simulink model "adaptivekoli"  (Simulink 7.1)
settings: Solver=ode45  StartTime=0.0  StopTime=100  RelTol=1e-3
InitFcn:
  | vo=502;
  | za=-1.01887*502;
  | zq=0.0949*502;
  | zd=-0.00215*502;
  | ma=0.82225;
  | mq=-1.07741;
  | md=-0.17555;
settings Model: Creator=zahra yaghoubi  LastModifiedBy=Yaghobi
settings OptimizationCC: InitFltsAndDblsToZero=off
settings DebuggingCC: StrictBusMsg=ErrorLevel1

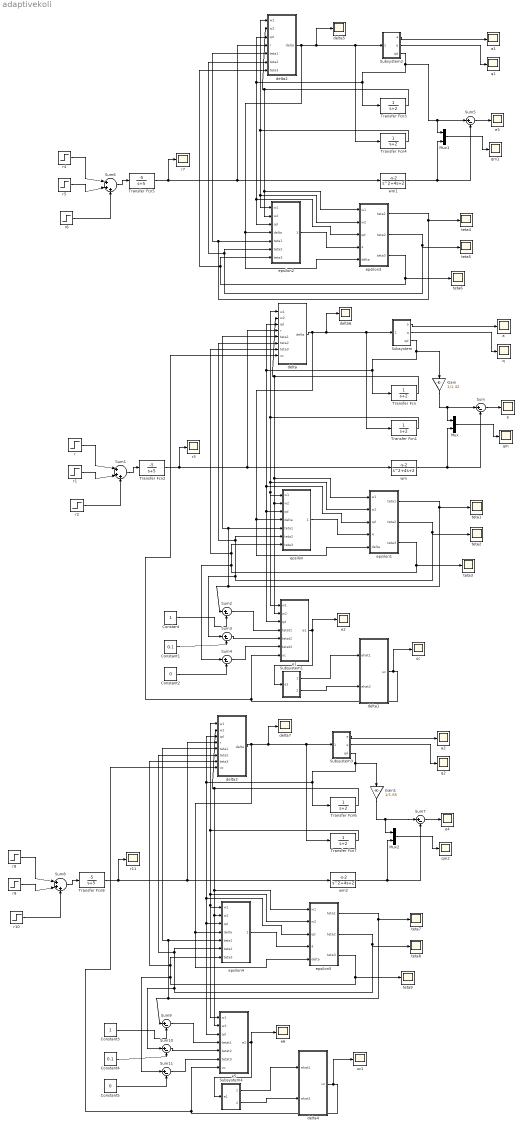
== system adaptivekoli ==
  Constant : Constant  OutDataType=sfix(16)  OutScaling=2^0
  Constant1 : Constant  Value=0.1  OutDataType=sfix(16)  OutScaling=2^0
  Constant2 : Constant  Value=0  OutDataType=sfix(16)  OutScaling=2^0
  Constant3 : Constant  OutDataType=sfix(16)  OutScaling=2^0
  Constant4 : Constant  Value=0.1  OutDataType=sfix(16)  OutScaling=2^0
  Constant5 : Constant  Value=0  OutDataType=sfix(16)  OutScaling=2^0
  Gain : Gain  Orientation=down  Gain=1/1.42  ParameterDataType=sfix(16)  ParameterScaling=2^0  OutDataType=sfix(16)  OutScaling=2^0
  Gain1 : Gain  Orientation=down  Gain=1/1.65  ParameterDataType=sfix(16)  ParameterScaling=2^0  OutDataType=sfix(16)  OutScaling=2^0
  Mux : Mux  Inputs=2
  Mux1 : Mux  Inputs=2
  Mux2 : Mux  Inputs=2
  Subsystem : Subsystem
  Subsystem1 : Subsystem
  Subsystem2 : Subsystem
  Subsystem3 : Subsystem
  Subsystem4 : Subsystem
  Sum{,2..5,7,9..11} (9 alike) : Sum  Inputs=|+-  OutDataType=sfix(16)  OutScaling=2^0
  Sum1 : Sum  Inputs=|+++  OutDataType=sfix(16)  OutScaling=2^0
  Sum6 : Sum  Inputs=|+++  OutDataType=sfix(16)  OutScaling=2^0
  Sum8 : Sum  Inputs=|+++  OutDataType=sfix(16)  OutScaling=2^0
  Transfer Fcn{,1,3..4,6..7} (6 alike) : TransferFcn  Denominator=[1 2]
  Transfer Fcn2 : TransferFcn  Numerator=[-5]  Denominator=[1 5]
  Transfer Fcn5 : TransferFcn  Numerator=[-5]  Denominator=[1 5]
  Transfer Fcn8 : TransferFcn  Numerator=[-5]  Denominator=[1 5]
  a : Scope
      settings: SaveName=a2  DataFormat=Array  MaxDataPoints=50000
  a1 : Scope
      settings: SaveName=a1  DataFormat=Array  MaxDataPoints=50000
  a2 : Scope
      settings: SaveName=a3  DataFormat=Array  MaxDataPoints=50000
  delta : Subsystem
  delta1 : Subsystem
  delta2 : Subsystem
  delta3 : Subsystem
  delta4 : Subsystem
  delta5 : Scope
      settings: SaveName=delta1  DataFormat=Array  MaxDataPoints=50000
  delta6 : Scope
      settings: SaveName=delta2  DataFormat=Array  MaxDataPoints=50000
  delta7 : Scope
      settings: SaveName=delta3  DataFormat=Array  MaxDataPoints=50000
  e{,2..4,6} (5 alike) : Scope
      e settings: SaveName=e2  DataFormat=Array  MaxDataPoints=50000
      e2 settings: MaxDataPoints=50000
      e3 settings: SaveName=e1  DataFormat=Array  MaxDataPoints=50000
      e4 settings: SaveName=e3  DataFormat=Array  MaxDataPoints=50000
      e6 settings: SaveName=ScopeData3  MaxDataPoints=50000
  e1 : Subsystem
  e5 : Subsystem
  epsilon : Subsystem
  epsilon1 : Subsystem
  epsilon2 : Subsystem
  epsilon3 : Subsystem
  epsilon4 : Subsystem
  epsilon5 : Subsystem
  q : Scope
      settings: SaveName=q2  DataFormat=Array  MaxDataPoints=50000
  q1 : Scope
      settings: SaveName=q1  DataFormat=Array  MaxDataPoints=50000
  q2 : Scope
      settings: SaveName=q3  DataFormat=Array  MaxDataPoints=50000
  qm : Scope
      settings: SaveName=qm2  DataFormat=Array  MaxDataPoints=500000
  qm1 : Scope
      settings: SaveName=qm1  DataFormat=Array  MaxDataPoints=500000
  qm2 : Scope
      settings: SaveName=qm3  DataFormat=Array  MaxDataPoints=50000
  r : Step  Time=0  After=-1  SampleTime=0
  r1 : Step  Time=20  After=3  SampleTime=0
  r10 : Step  Time=40  After=-6  SampleTime=0
  r11 : Scope
      settings: SaveName=ScopeData4
  r2 : Step  Time=40  After=-6  SampleTime=0
  r3 : Scope
      settings: SaveName=r  DataFormat=Array  MaxDataPoints=50000
  r4 : Step  Time=0  After=-1  SampleTime=0
  r5 : Step  Time=20  After=3  SampleTime=0
  r6 : Step  Time=40  After=-6  SampleTime=0
  r7 : Scope
      settings: SaveName=ScopeData2
  r8 : Step  Time=0  After=-1  SampleTime=0
  r9 : Step  Time=20  After=3  SampleTime=0
  teta{1..9} (9 alike) : Scope
      teta1 settings: TimeRange=60  YMin=0  YMax=2  SaveName=teta12  DataFormat=Array  MaxDataPoints=50000
      teta2 settings: SaveName=teta22  DataFormat=Array  MaxDataPoints=50000
      teta3 settings: SaveName=teta32  DataFormat=Array  MaxDataPoints=50000
      teta4 settings: SaveName=teta11  DataFormat=Array  MaxDataPoints=50000
      teta5 settings: SaveName=teta21  DataFormat=Array  MaxDataPoints=50000
      teta6 settings: SaveName=teta31  DataFormat=Array  MaxDataPoints=50000
      teta7 settings: TimeRange=60  YMin=0  YMax=2  SaveName=teta13  DataFormat=Array  MaxDataPoints=50000
      teta8 settings: SaveName=teta23  DataFormat=Array  MaxDataPoints=50000
      teta9 settings: SaveName=teta33  DataFormat=Array  MaxDataPoints=50000
  uc : Scope
      settings: SaveName=uc1  DataFormat=Array  MaxDataPoints=50000
  uc1 : Scope
      settings: SaveName=uc2  DataFormat=Array  MaxDataPoints=50000
  wm : TransferFcn  Numerator=[-1 -2]  Denominator="[1 4  2]"
  wm1 : TransferFcn  Numerator=[-1 -2]  Denominator="[1 4  2]"
  wm2 : TransferFcn  Numerator=[-1 -2]  Denominator="[1 4  2]"
  wires:
  Subsystem/1(a) -> a/1
  Subsystem/2(q) -> q/1
  Subsystem/3(qd) -> Transfer Fcn/1, delta/3(qd), epsilon1/3(qd), epsilon/3(qd), e1/3(qd), Gain/1
  delta/1(delta) -> epsilon/4(delta), epsilon1/5(delta), Subsystem/1(delta), Transfer Fcn1/1, delta6/1
  wm/1 -> Sum/2, Mux/2
  Transfer Fcn/1 -> delta/2(w2), epsilon1/1(w1), epsilon/2(w2), e1/2(w2)
  Transfer Fcn1/1 -> delta/1(w1), epsilon1/2(w2), epsilon/1(w1), e1/1(w1)
  epsilon/1(epsilon) -> epsilon1/4(epsilon)
  epsilon1/1(teta1) -> teta1/1, epsilon/5(teta1), delta/5(teta1), Sum2/1
  epsilon1/2(teta2) -> teta2/1, epsilon/6(teta2), delta/6(teta2), Sum3/1
  epsilon1/3(teta3) -> teta3/1, epsilon/7(teta3), delta/7(teta3), Sum4/1
  Sum/1 -> e/1
  r/1 -> Sum1/1
  r1/1 -> Sum1/2
  r2/1 -> Sum1/3
  Sum1/1 -> Transfer Fcn2/1
  Mux/1 -> qm/1
  e1/1(e1) -> Subsystem1/1(e1), e2/1
  Subsystem1/1(ehat1) -> delta1/1(ehat1)
  delta1/1(uc) -> e1/7(uc), delta/8(uc), uc/1
  Sum4/1 -> e1/6(tetat3)
  Sum3/1 -> e1/5(tetat2)
  Sum2/1 -> e1/4(tetat1)
  Constant/1 -> Sum2/2
  Constant1/1 -> Sum3/2
  Constant2/1 -> Sum4/2
  Subsystem1/2(ehat2) -> delta1/2(ehat2)
  Transfer Fcn2/1 -> wm/1, delta/4(r), r3/1
  Gain/1 -> Sum/1, Mux/1
  Subsystem2/1(a) -> a1/1
  Subsystem2/2(q) -> q1/1
  Subsystem2/3(qd) -> Transfer Fcn3/1, delta2/3(qd), epsilon2/3(qd), epsilon3/3(qd), Sum5/1, Mux1/1
  delta2/1(delta) -> epsilon2/4(delta), epsilon3/5(delta), Subsystem2/1(delta), Transfer Fcn4/1, delta5/1
  wm1/1 -> Sum5/2, Mux1/2
  Transfer Fcn3/1 -> delta2/2(w2), epsilon2/2(w2), epsilon3/1(w1)
  Transfer Fcn4/1 -> delta2/1(w1), epsilon2/1(w1), epsilon3/2(w2)
  epsilon2/1(epsilon) -> epsilon3/4(epsilon)
  epsilon3/1(teta1) -> epsilon2/5(teta1), delta2/5(teta1), teta4/1
  epsilon3/2(teta2) -> epsilon2/6(teta2), delta2/6(teta2), teta5/1
  epsilon3/3(teta3) -> epsilon2/7(teta3), delta2/7(teta3), teta6/1
  Sum5/1 -> e3/1
  r4/1 -> Sum6/1
  r5/1 -> Sum6/2
  r6/1 -> Sum6/3
  Sum6/1 -> Transfer Fcn5/1
  Transfer Fcn5/1 -> wm1/1, delta2/4(r), r7/1
  Mux1/1 -> qm1/1
  Subsystem3/1(a) -> a2/1
  Subsystem3/2(q) -> q2/1
  Subsystem3/3(qd) -> Transfer Fcn6/1, delta3/3(qd), epsilon5/3(qd), epsilon4/3(qd), e5/3(qd), Gain1/1
  delta3/1(delta) -> epsilon4/4(delta), epsilon5/5(delta), Subsystem3/1(delta), Transfer Fcn7/1, delta7/1
  wm2/1 -> Sum7/2, Mux2/2
  Transfer Fcn6/1 -> delta3/2(w2), epsilon5/1(w1), epsilon4/2(w2), e5/2(w2)
  Transfer Fcn7/1 -> delta3/1(w1), epsilon5/2(w2), epsilon4/1(w1), e5/1(w1)
  epsilon4/1(epsilon) -> epsilon5/4(epsilon)
  epsilon5/1(teta1) -> teta7/1, epsilon4/5(teta1), delta3/5(teta1), Sum9/1
  epsilon5/2(teta2) -> teta8/1, epsilon4/6(teta2), delta3/6(teta2), Sum10/1
  epsilon5/3(teta3) -> teta9/1, epsilon4/7(teta3), delta3/7(teta3), Sum11/1
  Sum7/1 -> e4/1
  r8/1 -> Sum8/1
  r9/1 -> Sum8/2
  r10/1 -> Sum8/3
  Sum8/1 -> Transfer Fcn8/1
  Mux2/1 -> qm2/1
  e5/1(e1) -> Subsystem4/1(e1), e6/1
  Subsystem4/1(ehat1) -> delta4/1(ehat1)
  delta4/1(uc) -> e5/7(uc), delta3/8(uc), uc1/1
  Sum11/1 -> e5/6(tetat3)
  Sum10/1 -> e5/5(tetat2)
  Sum9/1 -> e5/4(tetat1)
  Constant3/1 -> Sum9/2
  Constant4/1 -> Sum10/2
  Constant5/1 -> Sum11/2
  Subsystem4/2(ehat2) -> delta4/2(ehat2)
  Transfer Fcn8/1 -> wm2/1, delta3/4(r), r11/1
  Gain1/1 -> Sum7/1, Mux2/1

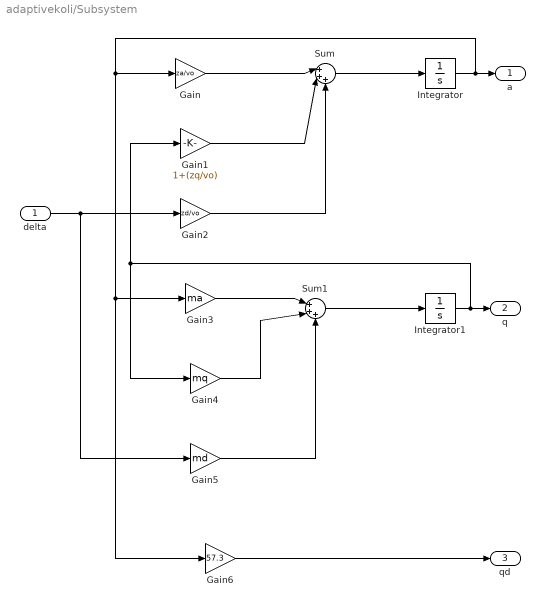
== system adaptivekoli/Subsystem ==
  delta : Inport
  Gain : Gain  Gain=za/vo  ParameterDataType=sfix(16)  ParameterScaling=2^0  OutDataType=sfix(16)  OutScaling=2^0
  Gain1 : Gain  Gain=1+(zq/vo)  ParameterDataType=sfix(16)  ParameterScaling=2^0  OutDataType=sfix(16)  OutScaling=2^0
  Gain2 : Gain  Gain=zd/vo  ParameterDataType=sfix(16)  ParameterScaling=2^0  OutDataType=sfix(16)  OutScaling=2^0
  Gain3 : Gain  Gain=ma  ParameterDataType=sfix(16)  ParameterScaling=2^0  OutDataType=sfix(16)  OutScaling=2^0
  Gain4 : Gain  Gain=mq  ParameterDataType=sfix(16)  ParameterScaling=2^0  OutDataType=sfix(16)  OutScaling=2^0
  Gain5 : Gain  Gain=md  ParameterDataType=sfix(16)  ParameterScaling=2^0  OutDataType=sfix(16)  OutScaling=2^0
  Gain6 : Gain  Gain=57.3  ParameterDataType=sfix(16)  ParameterScaling=2^0  OutDataType=sfix(16)  OutScaling=2^0
  Integrator : Integrator
  Integrator1 : Integrator
  Sum : Sum  Inputs=|+++  OutDataType=sfix(16)  OutScaling=2^0
  Sum1 : Sum  Inputs=|+++  OutDataType=sfix(16)  OutScaling=2^0
  a : Outport
  q : Outport  Port=2
  qd : Outport  Port=3
  wires:
  Integrator/1 -> Gain/1, Gain3/1, Gain6/1, a/1
  Gain/1 -> Sum/1
  Gain1/1 -> Sum/2
  Gain2/1 -> Sum/3
  Sum/1 -> Integrator/1
  Gain3/1 -> Sum1/1
  Gain4/1 -> Sum1/2
  Sum1/1 -> Integrator1/1
  Integrator1/1 -> Gain4/1, Gain1/1, q/1
  Gain5/1 -> Sum1/3
  delta/1 -> Gain2/1, Gain5/1
  Gain6/1 -> qd/1

== system adaptivekoli/Subsystem1 ==
  e1 : Inport
  Gain : Gain  Gain=-3.7375  ParameterDataType=sfix(16)  ParameterScaling=2^0  OutDataType=sfix(16)  OutScaling=2^0
  Gain1 : Gain  Gain=-0.8688  ParameterDataType=sfix(16)  ParameterScaling=2^0  OutDataType=sfix(16)  OutScaling=2^0
  Gain2 : Gain  Gain=0.7475  ParameterDataType=sfix(16)  ParameterScaling=2^0  OutDataType=sfix(16)  OutScaling=2^0
  Gain3 : Gain  Gain=-43.987  ParameterDataType=sfix(16)  ParameterScaling=2^0  OutDataType=sfix(16)  OutScaling=2^0
  Gain4 : Gain  Gain=-24.9851  ParameterDataType=sfix(16)  ParameterScaling=2^0  OutDataType=sfix(16)  OutScaling=2^0
  Gain5 : Gain  Gain=7.1710  ParameterDataType=sfix(16)  ParameterScaling=2^0  OutDataType=sfix(16)  OutScaling=2^0
  Integrator : Integrator
  Integrator1 : Integrator
  Sum : Sum  Inputs=|+++  OutDataType=sfix(16)  OutScaling=2^0
  Sum1 : Sum  Inputs=|+++  OutDataType=sfix(16)  OutScaling=2^0
  ehat1 : Outport
  ehat2 : Outport  Port=2
  wires:
  Integrator/1 -> Gain/1, Gain3/1, ehat1/1
  Gain/1 -> Sum/1
  Gain1/1 -> Sum/2
  Gain2/1 -> Sum/3
  Sum/1 -> Integrator/1
  Gain3/1 -> Sum1/1
  Gain4/1 -> Sum1/2
  Sum1/1 -> Integrator1/1
  Integrator1/1 -> Gain4/1, Gain1/1, ehat2/1
  Gain5/1 -> Sum1/3
  e1/1 -> Gain2/1, Gain5/1

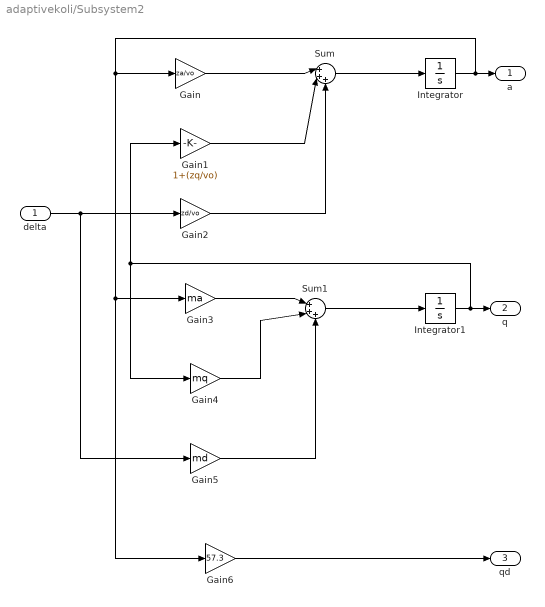
== system adaptivekoli/Subsystem2 ==
  delta : Inport
  Gain : Gain  Gain=za/vo  ParameterDataType=sfix(16)  ParameterScaling=2^0  OutDataType=sfix(16)  OutScaling=2^0
  Gain1 : Gain  Gain=1+(zq/vo)  ParameterDataType=sfix(16)  ParameterScaling=2^0  OutDataType=sfix(16)  OutScaling=2^0
  Gain2 : Gain  Gain=zd/vo  ParameterDataType=sfix(16)  ParameterScaling=2^0  OutDataType=sfix(16)  OutScaling=2^0
  Gain3 : Gain  Gain=ma  ParameterDataType=sfix(16)  ParameterScaling=2^0  OutDataType=sfix(16)  OutScaling=2^0
  Gain4 : Gain  Gain=mq  ParameterDataType=sfix(16)  ParameterScaling=2^0  OutDataType=sfix(16)  OutScaling=2^0
  Gain5 : Gain  Gain=md  ParameterDataType=sfix(16)  ParameterScaling=2^0  OutDataType=sfix(16)  OutScaling=2^0
  Gain6 : Gain  Gain=57.3  ParameterDataType=sfix(16)  ParameterScaling=2^0  OutDataType=sfix(16)  OutScaling=2^0
  Integrator : Integrator
  Integrator1 : Integrator
  Sum : Sum  Inputs=|+++  OutDataType=sfix(16)  OutScaling=2^0
  Sum1 : Sum  Inputs=|+++  OutDataType=sfix(16)  OutScaling=2^0
  a : Outport
  q : Outport  Port=2
  qd : Outport  Port=3
  wires:
  Integrator/1 -> Gain/1, Gain3/1, Gain6/1, a/1
  Gain/1 -> Sum/1
  Gain1/1 -> Sum/2
  Gain2/1 -> Sum/3
  Sum/1 -> Integrator/1
  Gain3/1 -> Sum1/1
  Gain4/1 -> Sum1/2
  Sum1/1 -> Integrator1/1
  Integrator1/1 -> Gain4/1, Gain1/1, q/1
  Gain5/1 -> Sum1/3
  delta/1 -> Gain2/1, Gain5/1
  Gain6/1 -> qd/1

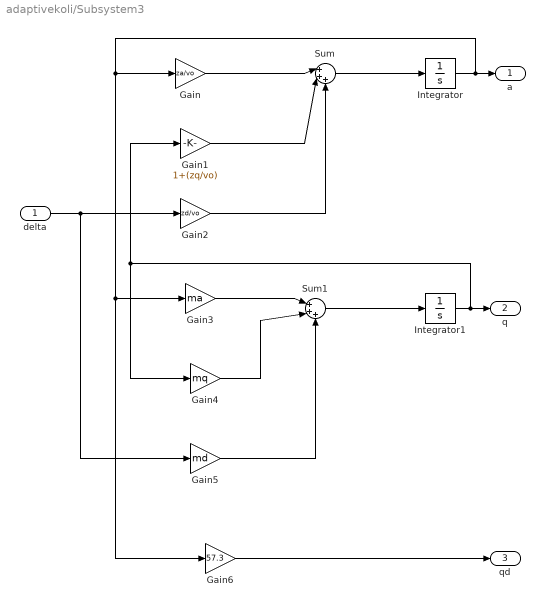
== system adaptivekoli/Subsystem3 ==
  delta : Inport
  Gain : Gain  Gain=za/vo  ParameterDataType=sfix(16)  ParameterScaling=2^0  OutDataType=sfix(16)  OutScaling=2^0
  Gain1 : Gain  Gain=1+(zq/vo)  ParameterDataType=sfix(16)  ParameterScaling=2^0  OutDataType=sfix(16)  OutScaling=2^0
  Gain2 : Gain  Gain=zd/vo  ParameterDataType=sfix(16)  ParameterScaling=2^0  OutDataType=sfix(16)  OutScaling=2^0
  Gain3 : Gain  Gain=ma  ParameterDataType=sfix(16)  ParameterScaling=2^0  OutDataType=sfix(16)  OutScaling=2^0
  Gain4 : Gain  Gain=mq  ParameterDataType=sfix(16)  ParameterScaling=2^0  OutDataType=sfix(16)  OutScaling=2^0
  Gain5 : Gain  Gain=md  ParameterDataType=sfix(16)  ParameterScaling=2^0  OutDataType=sfix(16)  OutScaling=2^0
  Gain6 : Gain  Gain=57.3  ParameterDataType=sfix(16)  ParameterScaling=2^0  OutDataType=sfix(16)  OutScaling=2^0
  Integrator : Integrator
  Integrator1 : Integrator
  Sum : Sum  Inputs=|+++  OutDataType=sfix(16)  OutScaling=2^0
  Sum1 : Sum  Inputs=|+++  OutDataType=sfix(16)  OutScaling=2^0
  a : Outport
  q : Outport  Port=2
  qd : Outport  Port=3
  wires:
  Integrator/1 -> Gain/1, Gain3/1, Gain6/1, a/1
  Gain/1 -> Sum/1
  Gain1/1 -> Sum/2
  Gain2/1 -> Sum/3
  Sum/1 -> Integrator/1
  Gain3/1 -> Sum1/1
  Gain4/1 -> Sum1/2
  Sum1/1 -> Integrator1/1
  Integrator1/1 -> Gain4/1, Gain1/1, q/1
  Gain5/1 -> Sum1/3
  delta/1 -> Gain2/1, Gain5/1
  Gain6/1 -> qd/1

== system adaptivekoli/Subsystem4 ==
  e1 : Inport
  Gain : Gain  Gain=-872.75  ParameterDataType=sfix(16)  ParameterScaling=2^0  OutDataType=sfix(16)  OutScaling=2^0
  Gain1 : Gain  Gain=-435.375  ParameterDataType=sfix(16)  ParameterScaling=2^0  OutDataType=sfix(16)  OutScaling=2^0
  Gain2 : Gain  Gain=174.55  ParameterDataType=sfix(16)  ParameterScaling=2^0  OutDataType=sfix(16)  OutScaling=2^0
  Gain3 : Gain  Gain=-269.304  ParameterDataType=sfix(16)  ParameterScaling=2^0  OutDataType=sfix(16)  OutScaling=2^0
  Gain4 : Gain  Gain=-137.252  ParameterDataType=sfix(16)  ParameterScaling=2^0  OutDataType=sfix(16)  OutScaling=2^0
  Gain5 : Gain  Gain=47  ParameterDataType=sfix(16)  ParameterScaling=2^0  OutDataType=sfix(16)  OutScaling=2^0
  Integrator : Integrator
  Integrator1 : Integrator
  Sum : Sum  Inputs=|+++  OutDataType=sfix(16)  OutScaling=2^0
  Sum1 : Sum  Inputs=|+++  OutDataType=sfix(16)  OutScaling=2^0
  ehat1 : Outport
  ehat2 : Outport  Port=2
  wires:
  Integrator/1 -> Gain/1, Gain3/1, ehat1/1
  Gain/1 -> Sum/1
  Gain1/1 -> Sum/2
  Gain2/1 -> Sum/3
  Sum/1 -> Integrator/1
  Gain3/1 -> Sum1/1
  Gain4/1 -> Sum1/2
  Sum1/1 -> Integrator1/1
  Integrator1/1 -> Gain4/1, Gain1/1, ehat2/1
  Gain5/1 -> Sum1/3
  e1/1 -> Gain2/1, Gain5/1

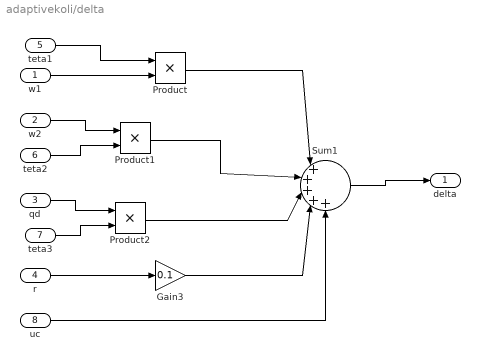
== system adaptivekoli/delta ==
  w1 : Inport
  w2 : Inport  Port=2
  qd : Inport  Port=3
  r : Inport  Port=4
  teta1 : Inport  Port=5
  teta2 : Inport  Port=6
  teta3 : Inport  Port=7
  uc : Inport  Port=8
  Gain3 : Gain  Gain=0.1  ParameterDataType=sfix(16)  ParameterScaling=2^0  OutDataType=sfix(16)  OutScaling=2^0
  Product : Product  OutDataType=sfix(16)  OutScaling=2^0  RndMeth=Zero
  Product1 : Product  OutDataType=sfix(16)  OutScaling=2^0  RndMeth=Zero
  Product2 : Product  OutDataType=sfix(16)  OutScaling=2^0  RndMeth=Zero
  Sum1 : Sum  Inputs=|+++++  OutDataType=sfix(16)  OutScaling=2^0
  delta : Outport
  wires:
  w1/1 -> Product/2
  r/1 -> Gain3/1
  teta1/1 -> Product/1
  w2/1 -> Product1/1
  teta2/1 -> Product1/2
  qd/1 -> Product2/1
  teta3/1 -> Product2/2
  Product/1 -> Sum1/1
  Product1/1 -> Sum1/2
  Product2/1 -> Sum1/3
  Gain3/1 -> Sum1/4
  Sum1/1 -> delta/1
  uc/1 -> Sum1/5

== system adaptivekoli/delta1 ==
  ehat1 : Inport
  ehat2 : Inport  Port=2
  Gain1 : Gain  Gain=0.7644  ParameterDataType=sfix(16)  ParameterScaling=2^0  OutDataType=sfix(16)  OutScaling=2^0
  Gain3 : Gain  Gain=1.533  ParameterDataType=sfix(16)  ParameterScaling=2^0  OutDataType=sfix(16)  OutScaling=2^0
  Sum1 : Sum  Inputs=|++  OutDataType=sfix(16)  OutScaling=2^0
  uc : Outport
  wires:
  ehat1/1 -> Gain3/1
  Gain3/1 -> Sum1/1
  Gain1/1 -> Sum1/2
  Sum1/1 -> uc/1
  ehat2/1 -> Gain1/1

== system adaptivekoli/delta2 ==
  w1 : Inport
  w2 : Inport  Port=2
  qd : Inport  Port=3
  r : Inport  Port=4
  teta1 : Inport  Port=5
  teta2 : Inport  Port=6
  teta3 : Inport  Port=7
  Gain3 : Gain  Gain=0.1  ParameterDataType=sfix(16)  ParameterScaling=2^0  OutDataType=sfix(16)  OutScaling=2^0
  Product : Product  OutDataType=sfix(16)  OutScaling=2^0  RndMeth=Zero
  Product1 : Product  OutDataType=sfix(16)  OutScaling=2^0  RndMeth=Zero
  Product2 : Product  OutDataType=sfix(16)  OutScaling=2^0  RndMeth=Zero
  Sum1 : Sum  Inputs=|++++  OutDataType=sfix(16)  OutScaling=2^0
  delta : Outport
  wires:
  w1/1 -> Product/2
  r/1 -> Gain3/1
  teta1/1 -> Product/1
  w2/1 -> Product1/1
  teta2/1 -> Product1/2
  qd/1 -> Product2/1
  teta3/1 -> Product2/2
  Product/1 -> Sum1/1
  Product1/1 -> Sum1/2
  Product2/1 -> Sum1/3
  Gain3/1 -> Sum1/4
  Sum1/1 -> delta/1

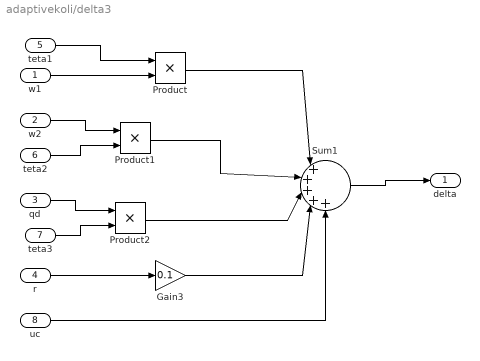
== system adaptivekoli/delta3 ==
  w1 : Inport
  w2 : Inport  Port=2
  qd : Inport  Port=3
  r : Inport  Port=4
  teta1 : Inport  Port=5
  teta2 : Inport  Port=6
  teta3 : Inport  Port=7
  uc : Inport  Port=8
  Gain3 : Gain  Gain=0.1  ParameterDataType=sfix(16)  ParameterScaling=2^0  OutDataType=sfix(16)  OutScaling=2^0
  Product : Product  OutDataType=sfix(16)  OutScaling=2^0  RndMeth=Zero
  Product1 : Product  OutDataType=sfix(16)  OutScaling=2^0  RndMeth=Zero
  Product2 : Product  OutDataType=sfix(16)  OutScaling=2^0  RndMeth=Zero
  Sum1 : Sum  Inputs=|+++++  OutDataType=sfix(16)  OutScaling=2^0
  delta : Outport
  wires:
  w1/1 -> Product/2
  r/1 -> Gain3/1
  teta1/1 -> Product/1
  w2/1 -> Product1/1
  teta2/1 -> Product1/2
  qd/1 -> Product2/1
  teta3/1 -> Product2/2
  Product/1 -> Sum1/1
  Product1/1 -> Sum1/2
  Product2/1 -> Sum1/3
  Gain3/1 -> Sum1/4
  Sum1/1 -> delta/1
  uc/1 -> Sum1/5

== system adaptivekoli/delta4 ==
  ehat1 : Inport
  ehat2 : Inport  Port=2
  Gain1 : Gain  Gain=3.938  ParameterDataType=sfix(16)  ParameterScaling=2^0  OutDataType=sfix(16)  OutScaling=2^0
  Gain3 : Gain  Gain=8.076  ParameterDataType=sfix(16)  ParameterScaling=2^0  OutDataType=sfix(16)  OutScaling=2^0
  Sum1 : Sum  Inputs=|++  OutDataType=sfix(16)  OutScaling=2^0
  uc : Outport
  wires:
  ehat1/1 -> Gain3/1
  Gain3/1 -> Sum1/1
  Gain1/1 -> Sum1/2
  Sum1/1 -> uc/1
  ehat2/1 -> Gain1/1

== system adaptivekoli/e1 ==
  w1 : Inport
  w2 : Inport  Port=2
  qd : Inport  Port=3
  tetat1 : Inport  Port=4
  tetat2 : Inport  Port=5
  tetat3 : Inport  Port=6
  uc : Inport  Port=7
  Product : Product  OutDataType=sfix(16)  OutScaling=2^0  RndMeth=Zero
  Product1 : Product  OutDataType=sfix(16)  OutScaling=2^0  RndMeth=Zero
  Product2 : Product  OutDataType=sfix(16)  OutScaling=2^0  RndMeth=Zero
  Sum1 : Sum  Inputs=|++++  OutDataType=sfix(16)  OutScaling=2^0
  wm : TransferFcn  Numerator=[-10 -20]  Denominator="[1 4  2]"
  e1 : Outport
  wires:
  w1/1 -> Product/2
  tetat1/1 -> Product/1
  w2/1 -> Product1/1
  tetat2/1 -> Product1/2
  qd/1 -> Product2/1
  tetat3/1 -> Product2/2
  Product/1 -> Sum1/1
  Product1/1 -> Sum1/2
  Product2/1 -> Sum1/3
  Sum1/1 -> wm/1
  uc/1 -> Sum1/4
  wm/1 -> e1/1

== system adaptivekoli/e5 ==
  w1 : Inport
  w2 : Inport  Port=2
  qd : Inport  Port=3
  tetat1 : Inport  Port=4
  tetat2 : Inport  Port=5
  tetat3 : Inport  Port=6
  uc : Inport  Port=7
  Product : Product  OutDataType=sfix(16)  OutScaling=2^0  RndMeth=Zero
  Product1 : Product  OutDataType=sfix(16)  OutScaling=2^0  RndMeth=Zero
  Product2 : Product  OutDataType=sfix(16)  OutScaling=2^0  RndMeth=Zero
  Sum1 : Sum  Inputs=|++++  OutDataType=sfix(16)  OutScaling=2^0
  wm : TransferFcn  Numerator=[-10 -20]  Denominator="[1 4  2]"
  e1 : Outport
  wires:
  w1/1 -> Product/2
  tetat1/1 -> Product/1
  w2/1 -> Product1/1
  tetat2/1 -> Product1/2
  qd/1 -> Product2/1
  tetat3/1 -> Product2/2
  Product/1 -> Sum1/1
  Product1/1 -> Sum1/2
  Product2/1 -> Sum1/3
  Sum1/1 -> wm/1
  uc/1 -> Sum1/4
  wm/1 -> e1/1

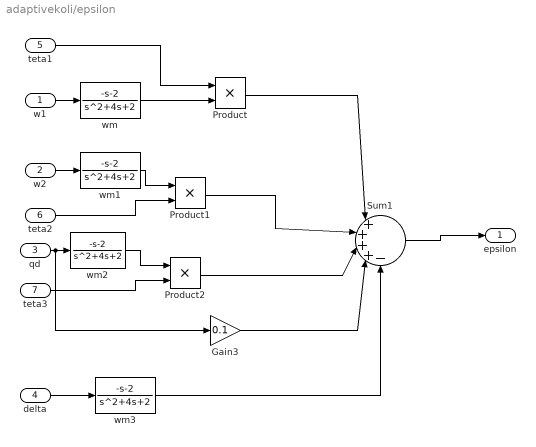
== system adaptivekoli/epsilon ==
  w1 : Inport
  w2 : Inport  Port=2
  qd : Inport  Port=3
  delta : Inport  Port=4
  teta1 : Inport  Port=5
  teta2 : Inport  Port=6
  teta3 : Inport  Port=7
  Gain3 : Gain  Gain=0.1  ParameterDataType=sfix(16)  ParameterScaling=2^0  OutDataType=sfix(16)  OutScaling=2^0
  Product : Product  OutDataType=sfix(16)  OutScaling=2^0  RndMeth=Zero
  Product1 : Product  OutDataType=sfix(16)  OutScaling=2^0  RndMeth=Zero
  Product2 : Product  OutDataType=sfix(16)  OutScaling=2^0  RndMeth=Zero
  Sum1 : Sum  Inputs=|++++-  OutDataType=sfix(16)  OutScaling=2^0
  wm{,1..3} (4 alike) : TransferFcn  Numerator=[-1 -2]  Denominator="[1 4  2]"
  epsilon : Outport
  wires:
  w1/1 -> wm/1
  teta1/1 -> Product/1
  w2/1 -> wm1/1
  teta2/1 -> Product1/2
  qd/1 -> wm2/1, Gain3/1
  teta3/1 -> Product2/2
  Product/1 -> Sum1/1
  Product1/1 -> Sum1/2
  Product2/1 -> Sum1/3
  Gain3/1 -> Sum1/4
  Sum1/1 -> epsilon/1
  wm/1 -> Product/2
  wm1/1 -> Product1/1
  wm2/1 -> Product2/1
  delta/1 -> wm3/1
  wm3/1 -> Sum1/5

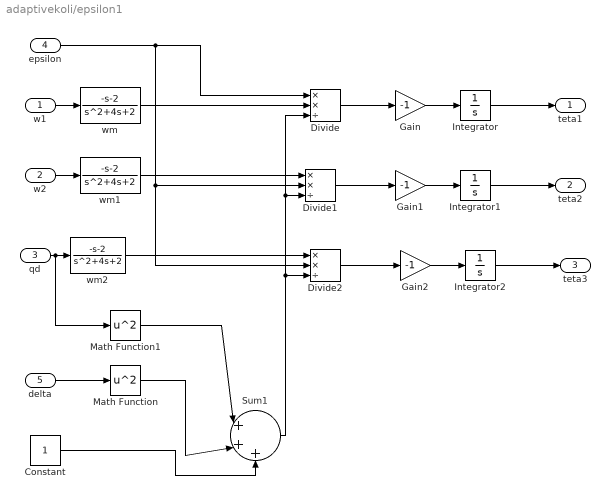
== system adaptivekoli/epsilon1 ==
  w1 : Inport
  w2 : Inport  Port=2
  qd : Inport  Port=3
  epsilon : Inport  Port=4
  delta : Inport  Port=5
  Constant : Constant  OutDataType=sfix(16)  OutScaling=2^0
  Divide : Product  Inputs=**/  OutDataType=sfix(16)  OutScaling=2^-10
  Divide1 : Product  Inputs=**/  OutDataType=sfix(16)  OutScaling=2^-10
  Divide2 : Product  Inputs=**/  OutDataType=sfix(16)  OutScaling=2^-10
  Gain : Gain  Gain=-1  ParameterDataType=sfix(16)  ParameterScaling=2^0  OutDataType=sfix(16)  OutScaling=2^0
  Gain1 : Gain  Gain=-1  ParameterDataType=sfix(16)  ParameterScaling=2^0  OutDataType=sfix(16)  OutScaling=2^0
  Gain2 : Gain  Gain=-1  ParameterDataType=sfix(16)  ParameterScaling=2^0  OutDataType=sfix(16)  OutScaling=2^0
  Integrator : Integrator  InitialCondition=1
  Integrator1 : Integrator  InitialCondition=.1
  Integrator2 : Integrator
  Math Function : Math  Operator=square  OutDataType=sfix(16)  OutScaling=2^0  SaturateOnIntegerOverflow=on
  Math Function1 : Math  Operator=square  OutDataType=sfix(16)  OutScaling=2^0  SaturateOnIntegerOverflow=on
  Sum1 : Sum  Inputs=|+++  OutDataType=sfix(16)  OutScaling=2^0
  wm : TransferFcn  Numerator=[-1 -2]  Denominator="[1 4  2]"
  wm1 : TransferFcn  Numerator=[-1 -2]  Denominator="[1 4  2]"
  wm2 : TransferFcn  Numerator=[-1 -2]  Denominator="[1 4  2]"
  teta1 : Outport
  teta2 : Outport  Port=2
  teta3 : Outport  Port=3
  wires:
  w1/1 -> wm/1
  w2/1 -> wm1/1
  qd/1 -> wm2/1, Math Function1/1
  wm/1 -> Divide/2
  wm1/1 -> Divide1/1
  wm2/1 -> Divide2/1
  epsilon/1 -> Divide/1, Divide1/2, Divide2/2
  delta/1 -> Math Function/1
  Math Function1/1 -> Sum1/1
  Math Function/1 -> Sum1/2
  Constant/1 -> Sum1/3
  Sum1/1 -> Divide/3, Divide1/3, Divide2/3
  Divide/1 -> Gain/1
  Gain/1 -> Integrator/1
  Integrator/1 -> teta1/1
  Divide1/1 -> Gain1/1
  Gain1/1 -> Integrator1/1
  Integrator1/1 -> teta2/1
  Divide2/1 -> Gain2/1
  Gain2/1 -> Integrator2/1
  Integrator2/1 -> teta3/1

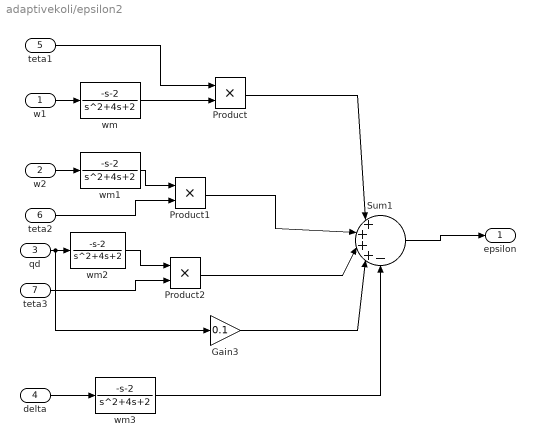
== system adaptivekoli/epsilon2 ==
  w1 : Inport
  w2 : Inport  Port=2
  qd : Inport  Port=3
  delta : Inport  Port=4
  teta1 : Inport  Port=5
  teta2 : Inport  Port=6
  teta3 : Inport  Port=7
  Gain3 : Gain  Gain=0.1  ParameterDataType=sfix(16)  ParameterScaling=2^0  OutDataType=sfix(16)  OutScaling=2^0
  Product : Product  OutDataType=sfix(16)  OutScaling=2^0  RndMeth=Zero
  Product1 : Product  OutDataType=sfix(16)  OutScaling=2^0  RndMeth=Zero
  Product2 : Product  OutDataType=sfix(16)  OutScaling=2^0  RndMeth=Zero
  Sum1 : Sum  Inputs=|++++-  OutDataType=sfix(16)  OutScaling=2^0
  wm{,1..3} (4 alike) : TransferFcn  Numerator=[-1 -2]  Denominator="[1 4  2]"
  epsilon : Outport
  wires:
  w1/1 -> wm/1
  teta1/1 -> Product/1
  w2/1 -> wm1/1
  teta2/1 -> Product1/2
  qd/1 -> wm2/1, Gain3/1
  teta3/1 -> Product2/2
  Product/1 -> Sum1/1
  Product1/1 -> Sum1/2
  Product2/1 -> Sum1/3
  Gain3/1 -> Sum1/4
  Sum1/1 -> epsilon/1
  wm/1 -> Product/2
  wm1/1 -> Product1/1
  wm2/1 -> Product2/1
  delta/1 -> wm3/1
  wm3/1 -> Sum1/5

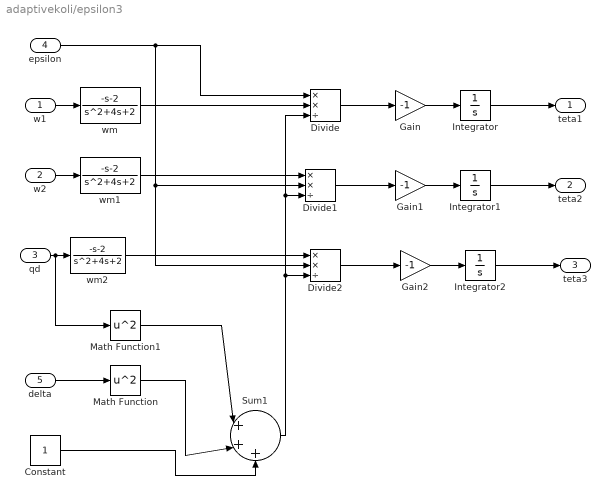
== system adaptivekoli/epsilon3 ==
  w1 : Inport
  w2 : Inport  Port=2
  qd : Inport  Port=3
  epsilon : Inport  Port=4
  delta : Inport  Port=5
  Constant : Constant  OutDataType=sfix(16)  OutScaling=2^0
  Divide : Product  Inputs=**/  OutDataType=sfix(16)  OutScaling=2^-10
  Divide1 : Product  Inputs=**/  OutDataType=sfix(16)  OutScaling=2^-10
  Divide2 : Product  Inputs=**/  OutDataType=sfix(16)  OutScaling=2^-10
  Gain : Gain  Gain=-1  ParameterDataType=sfix(16)  ParameterScaling=2^0  OutDataType=sfix(16)  OutScaling=2^0
  Gain1 : Gain  Gain=-1  ParameterDataType=sfix(16)  ParameterScaling=2^0  OutDataType=sfix(16)  OutScaling=2^0
  Gain2 : Gain  Gain=-1  ParameterDataType=sfix(16)  ParameterScaling=2^0  OutDataType=sfix(16)  OutScaling=2^0
  Integrator : Integrator  InitialCondition=1
  Integrator1 : Integrator  InitialCondition=.1
  Integrator2 : Integrator
  Math Function : Math  Operator=square  OutDataType=sfix(16)  OutScaling=2^0  SaturateOnIntegerOverflow=on
  Math Function1 : Math  Operator=square  OutDataType=sfix(16)  OutScaling=2^0  SaturateOnIntegerOverflow=on
  Sum1 : Sum  Inputs=|+++  OutDataType=sfix(16)  OutScaling=2^0
  wm : TransferFcn  Numerator=[-1 -2]  Denominator="[1 4  2]"
  wm1 : TransferFcn  Numerator=[-1 -2]  Denominator="[1 4  2]"
  wm2 : TransferFcn  Numerator=[-1 -2]  Denominator="[1 4  2]"
  teta1 : Outport
  teta2 : Outport  Port=2
  teta3 : Outport  Port=3
  wires:
  w1/1 -> wm/1
  w2/1 -> wm1/1
  qd/1 -> wm2/1, Math Function1/1
  wm/1 -> Divide/2
  wm1/1 -> Divide1/1
  wm2/1 -> Divide2/1
  epsilon/1 -> Divide/1, Divide1/2, Divide2/2
  delta/1 -> Math Function/1
  Math Function1/1 -> Sum1/1
  Math Function/1 -> Sum1/2
  Constant/1 -> Sum1/3
  Sum1/1 -> Divide/3, Divide1/3, Divide2/3
  Divide/1 -> Gain/1
  Gain/1 -> Integrator/1
  Integrator/1 -> teta1/1
  Divide1/1 -> Gain1/1
  Gain1/1 -> Integrator1/1
  Integrator1/1 -> teta2/1
  Divide2/1 -> Gain2/1
  Gain2/1 -> Integrator2/1
  Integrator2/1 -> teta3/1

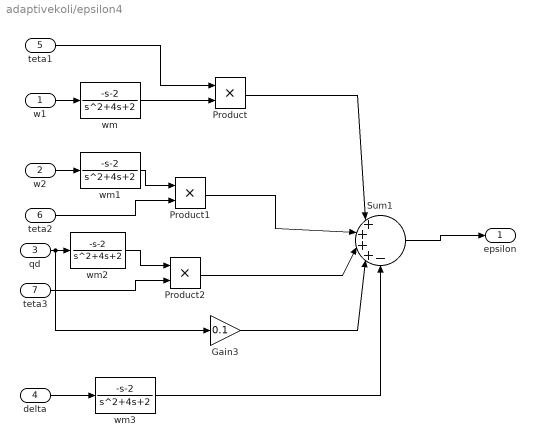
== system adaptivekoli/epsilon4 ==
  w1 : Inport
  w2 : Inport  Port=2
  qd : Inport  Port=3
  delta : Inport  Port=4
  teta1 : Inport  Port=5
  teta2 : Inport  Port=6
  teta3 : Inport  Port=7
  Gain3 : Gain  Gain=0.1  ParameterDataType=sfix(16)  ParameterScaling=2^0  OutDataType=sfix(16)  OutScaling=2^0
  Product : Product  OutDataType=sfix(16)  OutScaling=2^0  RndMeth=Zero
  Product1 : Product  OutDataType=sfix(16)  OutScaling=2^0  RndMeth=Zero
  Product2 : Product  OutDataType=sfix(16)  OutScaling=2^0  RndMeth=Zero
  Sum1 : Sum  Inputs=|++++-  OutDataType=sfix(16)  OutScaling=2^0
  wm{,1..3} (4 alike) : TransferFcn  Numerator=[-1 -2]  Denominator="[1 4  2]"
  epsilon : Outport
  wires:
  w1/1 -> wm/1
  teta1/1 -> Product/1
  w2/1 -> wm1/1
  teta2/1 -> Product1/2
  qd/1 -> wm2/1, Gain3/1
  teta3/1 -> Product2/2
  Product/1 -> Sum1/1
  Product1/1 -> Sum1/2
  Product2/1 -> Sum1/3
  Gain3/1 -> Sum1/4
  Sum1/1 -> epsilon/1
  wm/1 -> Product/2
  wm1/1 -> Product1/1
  wm2/1 -> Product2/1
  delta/1 -> wm3/1
  wm3/1 -> Sum1/5

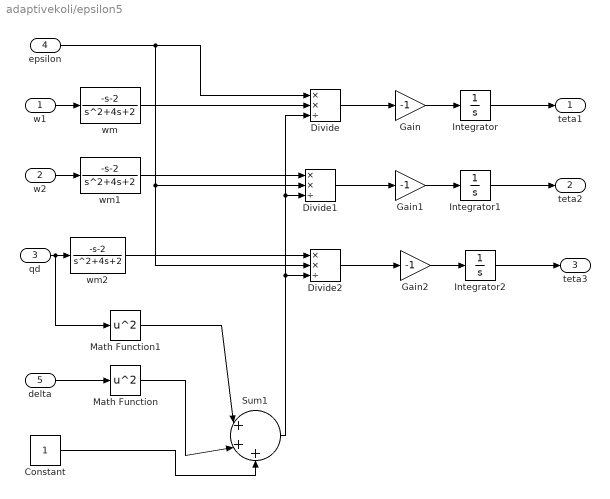
== system adaptivekoli/epsilon5 ==
  w1 : Inport
  w2 : Inport  Port=2
  qd : Inport  Port=3
  epsilon : Inport  Port=4
  delta : Inport  Port=5
  Constant : Constant  OutDataType=sfix(16)  OutScaling=2^0
  Divide : Product  Inputs=**/  OutDataType=sfix(16)  OutScaling=2^-10
  Divide1 : Product  Inputs=**/  OutDataType=sfix(16)  OutScaling=2^-10
  Divide2 : Product  Inputs=**/  OutDataType=sfix(16)  OutScaling=2^-10
  Gain : Gain  Gain=-1  ParameterDataType=sfix(16)  ParameterScaling=2^0  OutDataType=sfix(16)  OutScaling=2^0
  Gain1 : Gain  Gain=-1  ParameterDataType=sfix(16)  ParameterScaling=2^0  OutDataType=sfix(16)  OutScaling=2^0
  Gain2 : Gain  Gain=-1  ParameterDataType=sfix(16)  ParameterScaling=2^0  OutDataType=sfix(16)  OutScaling=2^0
  Integrator : Integrator  InitialCondition=1
  Integrator1 : Integrator  InitialCondition=.1
  Integrator2 : Integrator
  Math Function : Math  Operator=square  OutDataType=sfix(16)  OutScaling=2^0  SaturateOnIntegerOverflow=on
  Math Function1 : Math  Operator=square  OutDataType=sfix(16)  OutScaling=2^0  SaturateOnIntegerOverflow=on
  Sum1 : Sum  Inputs=|+++  OutDataType=sfix(16)  OutScaling=2^0
  wm : TransferFcn  Numerator=[-1 -2]  Denominator="[1 4  2]"
  wm1 : TransferFcn  Numerator=[-1 -2]  Denominator="[1 4  2]"
  wm2 : TransferFcn  Numerator=[-1 -2]  Denominator="[1 4  2]"
  teta1 : Outport
  teta2 : Outport  Port=2
  teta3 : Outport  Port=3
  wires:
  w1/1 -> wm/1
  w2/1 -> wm1/1
  qd/1 -> wm2/1, Math Function1/1
  wm/1 -> Divide/2
  wm1/1 -> Divide1/1
  wm2/1 -> Divide2/1
  epsilon/1 -> Divide/1, Divide1/2, Divide2/2
  delta/1 -> Math Function/1
  Math Function1/1 -> Sum1/1
  Math Function/1 -> Sum1/2
  Constant/1 -> Sum1/3
  Sum1/1 -> Divide/3, Divide1/3, Divide2/3
  Divide/1 -> Gain/1
  Gain/1 -> Integrator/1
  Integrator/1 -> teta1/1
  Divide1/1 -> Gain1/1
  Gain1/1 -> Integrator1/1
  Integrator1/1 -> teta2/1
  Divide2/1 -> Gain2/1
  Gain2/1 -> Integrator2/1
  Integrator2/1 -> teta3/1
